simulink model "drone_test_showcase"  (R2022a)
settings: Solver=VariableStepAuto  StartTime=0.0  StopTime=10  RelTol=1e-3
values from neighbouring files (symbols this model uses):
  D = [Env.UnrealRiverPts(Env.RiverRegions(i,4),1) Env.UnrealRiverPts(Env.RiverRegions(i,4),2)]    [DefineUAVPath.m]    (also in DistributeIceXML.m; DistributeIceXML1.m; DroneSurveyRegions.m; EstimateIceNumerals.m)
undefined symbols (not defined in the file or in its folder): Env
libraries: sim3dlib x8, visionsinks x3, sim3dcameralib x2, sim3dphyssensorlib x2, uavsim3dlib x2
settings Model: Creator=zckog  LastModifiedBy=zckog
settings DebuggingCC: UnconnectedInputMsg=warning  UnconnectedOutputMsg=warning  UnconnectedLineMsg=warning
settings RTWCC: DLArmComputeVersion=19.05

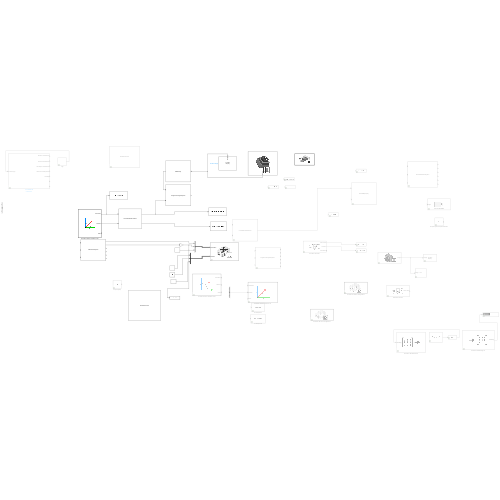
[thumbnail: Simulink's stored preview of the top-level diagram]
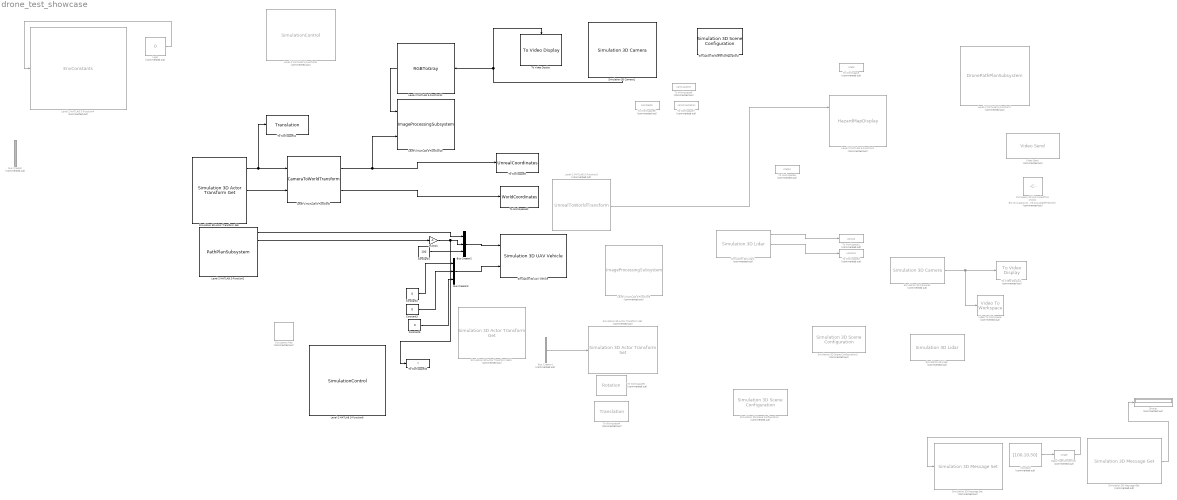
== system drone_test_showcase ==
  Bus Creator : BusCreator  Commented=on  Inputs=3
  Bus Creator1 : BusCreator  Commented=on  Inputs=3
  Bus Creator2 : BusCreator  Inputs=3
  Bus Creator3 : BusCreator  Inputs=3
  Constant : Constant  Commented=on  Value=[100,10,50]  VectorParams1D=off  OutDataTypeStr=single
  Constant1 : Constant  Value=100
  Constant2 : Constant  Value=0
  Constant3 : Constant  Value=0
  Constant5 : Constant  Value=0
  Data Type Conversion : DataTypeConversion  Commented=on  OutDataTypeStr=single  SaturateOnIntegerOverflow=off  RndMeth=Floor
  Display : Display  Commented=on
  Level-2 MATLAB S-Function1 : M-S-Function  Priority=1  Commented=on  FunctionName=HazardMapDisplay
  Level-2 MATLAB S-Function10 : M-S-Function  Priority=1  FunctionName=ImageProcessingSubsystem
  Level-2 MATLAB S-Function11 : M-S-Function  Priority=1  FunctionName=RGBToGray
  Level-2 MATLAB S-Function2 : M-S-Function  Priority=1  FunctionName=PathPlanSubsystem
  Level-2 MATLAB S-Function3 : M-S-Function  Priority=1  Commented=on  FunctionName=UnrealToWorldTransform
  Level-2 MATLAB S-Function4 : M-S-Function  Priority=1  Commented=on  FunctionName=EnvConstants
      mask Display:
      | port_label('input', 1, 'Control Logic');
      | port_label('output', 1, 'World to Unreal Tform');
      | port_label('output', 2, 'Unreal to World Tform');
      | port_label('output', 3, 'Occ Map to Unreal Tform');
      | port_label('output', 4, 'Unreal to Occ Map Tform');
      | port_label('output', 5, 'Occ Map');
  Level-2 MATLAB S-Function5 : M-S-Function  Priority=1  FunctionName=CameraToWorldTransform
  Level-2 MATLAB S-Function6 : M-S-Function  Priority=1  FunctionName=SimulationControl
  Level-2 MATLAB S-Function7 : M-S-Function  Priority=1  Commented=on  FunctionName=DronePathPlanSubsystem
  Level-2 MATLAB S-Function8 : M-S-Function  Priority=1  Commented=on  FunctionName=SimulationControl
  Level-2 MATLAB S-Function9 : M-S-Function  Priority=1  Commented=on  FunctionName=ImageProcessingSubsystem
  Logic : Constant  Commented=on  Value=0  OutDataTypeStr=double
  Multiply : Gain  Gain=-1
  OccupancyGrid-OccpiedThreshold1 : Constant  Commented=on  Value=Env.OccupancyGrid.OccupiedThreshold
  OccupancyMap : Constant  Commented=on  Value=Env.OccupancyMap
  Simulation 3D Actor Transform Get : sim3dlib/Simulation 3D Actor Transform Get  Priority=0  ActorTag=Drone1  NumberOfParts=1  CustNumOfParts=3  Ts=-1  aMode=2
      settings: SourceProductBaseCode=VE,AE,DR,UV,VE
  Simulation 3D Actor Transform Get1 : sim3dlib/Simulation 3D Actor Transform Get  Priority=0  Commented=on  ActorTag=SimulinkActor1  NumberOfParts=1  CustNumOfParts=3  Ts=-1  aMode=2
      settings: SourceProductBaseCode=VE,AE,DR,UV,VE
  Simulation 3D Actor Transform Set : sim3dlib/Simulation 3D Actor Transform Set  Priority=2  Commented=on  ActorTag=SimulinkActor1  NumberOfParts=1  CustNumOfParts=3  Translation=[0 0 0]  Rotation=[0 0 0]  Scale=[1 1 1]  Ts=-1  aMode=0
      settings: SourceProductBaseCode=VE,AE,DR,UV,VE
  Simulation 3D Camera1 : sim3dcameralib/Simulation 3D Camera  Priority=1  sensorTag=Sim3dSensor4  sensorId=4  sensorName=Sim3dSensor4  vehTagList={'Drone1';'Scene Origin'}  vehTag=Drone1  mountLoc=Origin  offsetFlag=on  tmountOffset=[0, 0, 0]  extTmount=off  rmountOffset=[0, 90, 90]  extRmount=off  FocalLength=[1109, 1109]  OpticalCenter=[640, 360]  ImageSize=[720, 1280]  RadialDistortion=[0, 0]  TangentialDistortion=[0, 0]  SensorSkew=0  DepthOutportEnabled=off  SemanticOutportEnabled=off  TransformOutportEnabled=off  SampleTime=-1  mountPoint=[0 0 0]  mountOrientation=[0 -90 -90]  aMode=3  ID=4
      settings: SourceProductBaseCode=VE,AE,DR,UV,VE
  Simulation 3D Camera2 : sim3dcameralib/Simulation 3D Camera  Priority=1  Commented=on  sensorTag=Sim3dSensor5  sensorId=5  sensorName=Sim3dSensor5  vehTagList={'Scene Origin';'SimulinkVehicle1'}  vehTag=SimulinkVehicle1  mountLoc=Origin  offsetFlag=on  tmountOffset=[0, 0, 0]  extTmount=off  rmountOffset=[0,45, 0]  extRmount=off  FocalLength=[1109, 1109]  OpticalCenter=[640, 360]  ImageSize=[720, 1280]  RadialDistortion=[0, 0]  TangentialDistortion=[0, 0]  SensorSkew=0  DepthOutportEnabled=off  SemanticOutportEnabled=off  TransformOutportEnabled=off  SampleTime=-1  mountPoint=[0 0 0]  mountOrientation=[0 -45 0]  aMode=3  ID=5
      settings: SourceProductBaseCode=VE,AE,DR,UV,VE
  Simulation 3D Lidar : sim3dphyssensorlib/Simulation 3D Lidar  Priority=1  Commented=on  sensorTag=Sim3dSensor2  sensorId=2  sensorName=Sim3dSensor2  vehTagList={'Scene Origin';'SimulinkVehicle1'}  vehTag=SimulinkVehicle1  mountLoc=Origin  offsetFlag=on  tmountOffset=[0, 0, 0]  rmountOffset=[0, 0, 0]  DetectionRange=120  RangeResolution=0.002  VerticalFOV=40  VerticalResolution=1.25  HorizontalFOV=360  HorizontalResolution=0.16  DistanceOutportEnabled=off  ReflectivityOutportEnabled=off  TransformOutportEnabled=off  SampleTime=-1  mountPoint=[0 0 0]  mountOrientation=[0 0 0]  aMode=4  ID=2
      settings: SourceProductBaseCode=VE,AE,DR,UV,VE
  Simulation 3D Lidar1 : sim3dphyssensorlib/Simulation 3D Lidar  Priority=1  Commented=on  sensorTag=Sim3dSensor3  sensorId=3  sensorName=Sim3dSensor3  vehTagList={'Scene Origin';'SimulinkVehicle1'}  vehTag=SimulinkVehicle1  mountLoc=Origin  offsetFlag=on  tmountOffset=[0, 0, 0]  rmountOffset=[0, 90,90]  DetectionRange=120  RangeResolution=0.002  VerticalFOV=40  VerticalResolution=1.25  HorizontalFOV=60  HorizontalResolution=0.16  DistanceOutportEnabled=off  ReflectivityOutportEnabled=off  TransformOutportEnabled=on  SampleTime=-1  mountPoint=[0 0 0]  mountOrientation=[0 -90 -90]  aMode=4  ID=3
      settings: SourceProductBaseCode=VE,AE,DR,UV,VE
  Simulation 3D Message Get : sim3dlib/Simulation 3D Message Get  Priority=1  Commented=on  SigName=ConeLocGet  DataType=single  MsgSize=[1 3]  Ts=-1  aMode=0
      settings: SourceProductBaseCode=VE,AE,DR,UV,VE
  Simulation 3D Message Set : sim3dlib/Simulation 3D Message Set  Priority=-1  Commented=on  SigName=ConeLocSet  Ts=-1  aMode=0
      settings: SourceProductBaseCode=VE,AE,DR,UV,VE
  Simulation 3D Scene Configuration : sim3dlib/Simulation 3D Scene Configuration  Priority=0  Commented=on  ProjectFormat=Unreal Editor  SceneDesc=US city block  ProjectName=D:\Matlab2021\toolbox\shared\sim3d_projects\automotive_project\UE4\WindowsNoEditor\VehicleSimulation.exe  ScenePath=/Game/Maps/USCityBlock  UEProjPath=C:\Users\noahvukosa\OneDrive - York University\Documents\DryLandscape\DryLandscape.uproject  vehTagList={'Scene Origin';'SimulinkVehicle1'}  vehTag=SimulinkVehicle1  OpVisEn=off  Ts=1/60  EnableWindow=on  EnableRemoteAccess=off  EnableWeather=off  SunAltitude=40.0  SunAzimuth=90  clouds=10  wind=1  fog=0  rain=0  sensorTag=MainCamera1  sensorId=1  sensorName=MainCamera1  mountLoc=Origin  offsetFlag=off  tmountOffset=[0, 0, 0]  rmountOffset=[0, 0, 0]  HorizontalResolution=1280  VerticalResolution=720  HorizontalFOV=60  mountPoint=[0 0 0]  mountOrientation=[0 0 0]  aMode=4  ID=1
      settings: SourceProductBaseCode=VE,AE,DR,UV,VE
  Simulation 3D Scene Configuration1 : sim3dlib/Simulation 3D Scene Configuration  Priority=0  Commented=on  ProjectFormat=Unreal Executable  SceneDesc=US city block  ProjectName=D:\OneDrive - York University\Unreal Projects\DryLandscape\Content\WindowsNoEditor\DryLandscape\Binaries\Win64\DryLandscape.exe  ScenePath=/Game/Maps/HwStrght  vehTagList={'Scene Origin';'SimulinkVehicle1'}  vehTag=SimulinkVehicle1  OpVisEn=off  Ts=1/60  EnableWindow=on  EnableRemoteAccess=off  EnableWeather=off  SunAltitude=40.0  SunAzimuth=90  clouds=10  wind=1  fog=0  rain=0  sensorTag=MainCamera2  sensorId=2  sensorName=MainCamera2  mountLoc=Origin  offsetFlag=off  tmountOffset=[0, 0, 0]  rmountOffset=[0, 0, 0]  HorizontalResolution=1280  VerticalResolution=720  HorizontalFOV=60  mountPoint=[0 0 0]  mountOrientation=[0 0 0]  aMode=4  ID=2
      settings: SourceProductBaseCode=VE,AE,DR,UV,VE
  Simulation 3D Scene Configuration2 : sim3dlib/Simulation 3D Scene Configuration  Priority=1  ProjectFormat=Unreal Editor  SceneDesc=Straight road  ProjectName=D:\Matlab2021\toolbox\shared\sim3d_projects\automotive_project\UE4\WindowsNoEditor\VehicleSimulation.exe  ScenePath=/Game/Maps/HwStrght  UEProjPath=D:\Personal Archives\OneDrive - York University\MASS\UNREALxMATLAB\UNREALxMATLAB\DroneExp1\DroneExp1\DroneExp1.uproject  vehTagList={'Scene Origin';'SimulinkVehicle1'}  vehTag=Scene Origin  OpVisEn=off  Ts=1/30  EnableWindow=on  EnableRemoteAccess=off  EnableWeather=off  SunAltitude=40.0  SunAzimuth=90  clouds=10  wind=1  fog=0  rain=0  sensorTag=MainCamera3  sensorId=3  sensorName=MainCamera3  mountLoc=Origin  offsetFlag=off  tmountOffset=[0, 0, 0]  rmountOffset=[0, 0, 0]  HorizontalResolution=1280  VerticalResolution=720  HorizontalFOV=60  mountPoint=[0 0 0]  mountOrientation=[0 0 0]  aMode=3  ID=3
      settings: SourceProductBaseCode=VE,AE,DR,UV,VE
  Simulation 3D UAV Vehicle : uavsim3dlib/Simulation 3D UAV Vehicle  Priority=2  Mesh=Quadrotor  MeshPath=/MathWorksUAVContent/UAVs/HexaRotorUAV/HexaRotor.HexaRotor  Color=Black  ActorName=Drone1  InitialTranslation=[0 0 0]  InitialRotation=[0 0 0]  SampleTime=-1  ActorType=SimulinkVehicle  ID=C  aMode=4  ActorTag=Drone1
      settings: SourceProductBaseCode=UV
  To Video Display : visionsinks/To Video Display  windowSizeMode=Normal  openAtMdlStart=on  fullScreen=off  videoWindowX=-1919  videoWindowY=31  saveWindowSize=off  videoWindowWidth=958  videoWindowHeight=1000  inputColorFormat=RGB  inputType=Obsolete  imagePorts=One multidimensional signal  OutputDevice=On-screen video monitor  dataOrg=Column-major  isWindowOpen=off
  To Video Display1 : visionsinks/To Video Display  Commented=on  windowSizeMode=Normal  openAtMdlStart=on  fullScreen=off  videoWindowX=61  videoWindowY=182  saveWindowSize=off  videoWindowWidth=1274  videoWindowHeight=460  inputColorFormat=RGB  inputType=Obsolete  imagePorts=One multidimensional signal  OutputDevice=On-screen video monitor  dataOrg=Column-major  isWindowOpen=off
  To Workspace : ToWorkspace  Commented=on  VariableName=state  SampleTime=-1
  To Workspace1 : ToWorkspace  Commented=on  VariableName=pCloud  SaveFormat=Timeseries  SampleTime=-1
  To Workspace10 : ToWorkspace  VariableName=Y  SaveFormat=Timeseries  SampleTime=-1
  To Workspace11 : ToWorkspace  VariableName=Translation  SaveFormat=Timeseries  SampleTime=-1
  To Workspace12 : ToWorkspace  VariableName=WorldCoordinates  SaveFormat=Timeseries  SampleTime=-1
  To Workspace2 : ToWorkspace  Commented=on  VariableName=Location  SaveFormat=Timeseries  SampleTime=-1
  To Workspace3 : ToWorkspace  VariableName=UnrealCoordinates  SaveFormat=Timeseries  SampleTime=-1
  To Workspace4 : ToWorkspace  Commented=on  VariableName=Translation  SampleTime=-1
      settings: Save2DSignal=2-D array (concatenate along first dimension)
  To Workspace5 : ToWorkspace  Commented=on  VariableName=Rotation  SampleTime=-1
      settings: Save2DSignal=2-D array (concatenate along first dimension)
  To Workspace6 : ToWorkspace  Commented=on  VariableName=camLocation  SaveFormat=Timeseries  SampleTime=-1
  To Workspace7 : ToWorkspace  Commented=on  VariableName=camOrientation  SaveFormat=Timeseries  SampleTime=-1
  To Workspace8 : ToWorkspace  Commented=on  VariableName=camDepth  SaveFormat=Timeseries  SampleTime=-1
  To Workspace9 : ToWorkspace  Commented=on  VariableName=state1  SampleTime=-1
  Video Send : uavsim3dlib/Video Send  Commented=on  ImageFormat=RGB  ImageSignal=One multidimensional signal  Compression=JPEG  JPEGQuality=85  VPXFrameDeadline=30  RemoteAddress=10.0.0.136  RemotePort=5004
      settings: SourceProductBaseCode=UV
  Video To Workspace : visionsinks/Video To Workspace  Commented=on  VariableName=vout  NumInputs=1  DataLimit=10  DecimationFactor=1  LogFi=off  InPortLabels=R|G|B
      settings: SourceProductBaseCode=VP
  wires:
  Constant/1 -> Data Type Conversion/1
  Data Type Conversion/1 -> Simulation 3D Message Set/1
  Simulation 3D Message Get/1 -> Display/1
  Simulation 3D Lidar1/1 -> To Workspace1/1
  Simulation 3D Lidar1/2 -> To Workspace2/1
  Simulation 3D Camera1/1 -> Level-2 MATLAB S-Function11/1, To Video Display/1
  Simulation 3D Camera2/1 -> Video To Workspace/1, To Video Display1/1
  Bus Creator1/1 -> Simulation 3D Actor Transform Set/2
  Constant1/1 -> Bus Creator2/3
  Bus Creator2/1 -> Simulation 3D UAV Vehicle/1
  Bus Creator3/1 -> Simulation 3D UAV Vehicle/2
  Level-2 MATLAB S-Function3/1 -> Level-2 MATLAB S-Function1/1
  Logic/1 -> Level-2 MATLAB S-Function4/1
  Constant2/1 -> Bus Creator3/1
  Constant3/1 -> Bus Creator3/2
  Multiply/1 -> Bus Creator2/2, To Workspace10/1
  Constant5/1 -> Bus Creator3/3
  Level-2 MATLAB S-Function2/1 -> Bus Creator2/1
  Level-2 MATLAB S-Function2/2 -> Multiply/1
  Level-2 MATLAB S-Function11/1 -> Level-2 MATLAB S-Function10/1
  Simulation 3D Actor Transform Get/1 -> To Workspace11/1, Level-2 MATLAB S-Function5/1
  Simulation 3D Actor Transform Get/2 -> Level-2 MATLAB S-Function5/2
  Level-2 MATLAB S-Function5/2 -> To Workspace12/1
  Level-2 MATLAB S-Function5/1 -> Level-2 MATLAB S-Function10/2, To Workspace3/1
